simulink model "rigid_body_fdyn_rotmat_test_com"  (Simulink 8.5)
settings: Solver=ode4  StartTime=0.0  StopTime=0.01  FixedStep=1.000000e-04  RelTol=1e-3
undefined symbols (not defined in the file or in its folder): g_W, I_B_C, m, r_B_B_C
undefined symbols (not defined in the file): DynPar1, KinPar_mdh
libraries: lib_rigid_body_dynamics x3, lib_rigid_body_kinematics x3, lib_transformations x2, vrlib x1
settings Model: Creator=schappler  LastModifiedBy=schappler
settings DataIOCC: LimitDataPoints=off  SaveFormat=StructureWithTime  SignalLoggingSaveFormat=Dataset
settings OptimizationCC: ExpressionDepthLimit=128
settings DebuggingCC: UnderspecifiedInitializationDetection=Simplified  MergeDetectMultiDrivingBlocksExec=error  FcnCallInpInsideContextMsg=EnableAllAsError  StateNameClashWarn=none
settings GRTTargetCC: CombineOutputUpdateFcns=on  GRTInterface=off

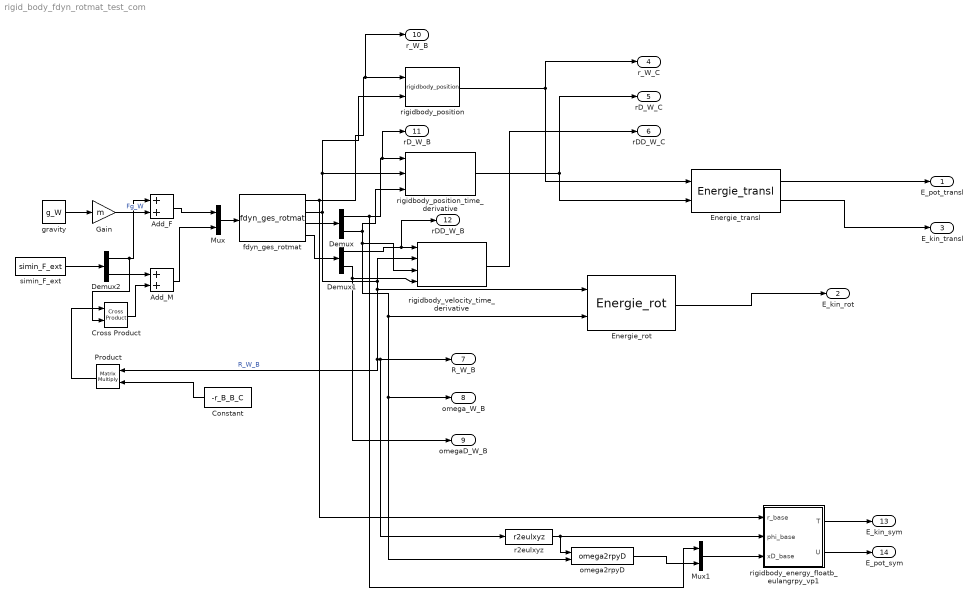
== system rigid_body_fdyn_rotmat_test_com ==
  Add_F : Sum
  Add_M : Sum
  Constant : Constant  Value=-r_B_B_C
  Cross Product : vrlib/Utilities/Cross Product
  Demux : Demux  Outputs=[3 3]
  Demux1 : Demux  Outputs=[3 3]
  Demux2 : Demux  Outputs=[3 3]
  Energie_rot : lib_rigid_body_dynamics/Energie_rot  I_B_C=I_B_C
  Energie_transl : lib_rigid_body_dynamics/Energie_transl  m=m  g_W=g_W
  Gain : Gain  Gain=m
  Mux : Mux  Inputs=2
  Mux1 : Mux  Inputs=2
  Product : Product  Multiplication=Matrix(*)
  r2eulxyz : lib_transformations/r2eulxyz
  fdyn_ges_rotmat : lib_rigid_body_dynamics/fdyn_ges_rotmat  I=I_B_C  m=m  r0=r0  rD0=rD0  R_t0=R_W_B_t0  omega0_t0=omega0_t0  r_B_B_C=r_B_B_C
  gravity : Constant  Value=g_W
  omega2rpyD : lib_transformations/omega2rpyD
  rigidbody_energy_floatb_eulangrpy_vp1 : Subsystem  mask{KinPar_mdh=KinPar_mdh, DynPar1=DynPar1, g_world=g_W}
      mask prompts: KinPar_mdh "Kinematik-Parameter"; DynPar1 "Dynamik-Parameter (Parametersatz 1)"; g_world "Gravitationsvektor im Welt-KS (g_world)"
  rigidbody_position : lib_rigid_body_kinematics/rigidbody_position  r_B_B_C=r_B_B_C  PktName_B='B'  PktName_C='C'
  rigidbody_position_time_derivative : lib_rigid_body_kinematics/rigidbody_position_time_derivative  r_B_B_C=r_B_B_C  PktName_B='B'  PktName_C='C'
  rigidbody_velocity_time_derivative : lib_rigid_body_kinematics/rigidbody_velocity_time_derivative  r_B_B_C=r_B_B_C  PktName_B='B'  PktName_C='C'
  simin_F_ext : FromWorkspace  VariableName=simin_F_ext  SampleTime=0  Interpolate=off  OutputAfterFinalValue=Holding final value
  E_pot_transl : Outport
  E_kin_rot : Outport  Port=2
  E_kin_transl : Outport  Port=3
  r_W_C : Outport  Port=4
  rD_W_C : Outport  Port=5
  rDD_W_C : Outport  Port=6
  R_W_B : Outport  Port=7
  omega_W_B : Outport  Port=8
  omegaD_W_B : Outport  Port=9
  r_W_B : Outport  Port=10
  rD_W_B : Outport  Port=11
  rDD_W_B : Outport  Port=12
  E_kin_sym : Outport  Port=13
  E_pot_sym : Outport  Port=14
  wires:
  gravity/1 -> Gain/1
  fdyn_ges_rotmat/2 -> rigidbody_position_time_derivative/2, rigidbody_position/2, rigidbody_velocity_time_derivative/2, Energie_rot/1, Product/1, r2eulxyz/1, R_W_B/1  "R_W_B"
  rigidbody_position/1 -> Energie_transl/1, r_W_C/1
  rigidbody_position_time_derivative/1 -> Energie_transl/2, rD_W_C/1
  Demux/2 -> rigidbody_position_time_derivative/3, rigidbody_velocity_time_derivative/3, Energie_rot/2, omega2rpyD/2, omega_W_B/1
  rigidbody_velocity_time_derivative/1 -> rDD_W_C/1
  Demux1/2 -> rigidbody_velocity_time_derivative/4, omegaD_W_B/1
  Energie_transl/1 -> E_pot_transl/1
  Energie_transl/2 -> E_kin_transl/1
  Energie_rot/1 -> E_kin_rot/1
  Gain/1 -> Add_F/2  "Fg_W"
  Mux/1 -> fdyn_ges_rotmat/1
  fdyn_ges_rotmat/3 -> Demux/1
  fdyn_ges_rotmat/1 -> rigidbody_energy_floatb_eulangrpy_vp1/1(r_base), rigidbody_position/1, r_W_B/1
  Demux/1 -> Mux1/1, rD_W_B/1, rigidbody_position_time_derivative/1
  fdyn_ges_rotmat/4 -> Demux1/1
  Demux1/1 -> rDD_W_B/1, rigidbody_velocity_time_derivative/1
  rigidbody_energy_floatb_eulangrpy_vp1/1(T) -> E_kin_sym/1
  rigidbody_energy_floatb_eulangrpy_vp1/2(U) -> E_pot_sym/1
  r2eulxyz/1 -> omega2rpyD/1, rigidbody_energy_floatb_eulangrpy_vp1/2(phi_base)
  omega2rpyD/1 -> Mux1/2
  Mux1/1 -> rigidbody_energy_floatb_eulangrpy_vp1/3(xD_base)
  simin_F_ext/1 -> Demux2/1
  Demux2/1 -> Cross Product/2, Add_F/1
  Demux2/2 -> Add_M/1
  Add_F/1 -> Mux/1
  Constant/1 -> Product/2
  Product/1 -> Cross Product/1
  Cross Product/1 -> Add_M/2
  Add_M/1 -> Mux/2

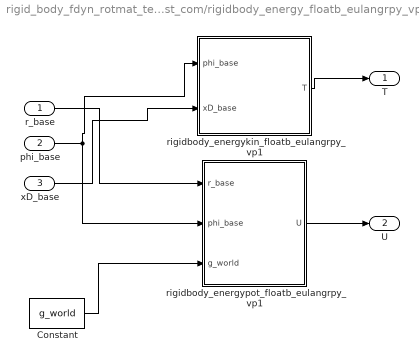
== system rigid_body_fdyn_rotmat_test_com/rigidbody_energy_floatb_eulangrpy_vp1 ==
  r_base : Inport
  phi_base : Inport  Port=2
  xD_base : Inport  Port=3
  Constant : Constant  Value=g_world
  rigidbody_energykin_floatb_eulangrpy_vp1 : Subsystem  mask{KinPar_mdh=KinPar_mdh, DynPar1=DynPar1}
      mask prompts: KinPar_mdh "Kinematik-Parameter"; DynPar1 "Dynamik-Parameter (Parametersatz 1)"
      mask init:
      | a_mdh = KinPar_mdh.a;
      | d_mdh = KinPar_mdh.d;
      | b_mdh = KinPar_mdh.b;
      | beta_mdh = KinPar_mdh.beta;
      | alpha_mdh = KinPar_mdh.alpha;
      | q_offset_mdh = KinPar_mdh.q_offset;
      | 
      | m = DynPar1.m;
      | r_S = DynPar1.r_S;
      | I_S = DynPar1.I_S;
  rigidbody_energypot_floatb_eulangrpy_vp1 : Subsystem  mask{KinPar_mdh=KinPar_mdh, DynPar1=DynPar1}
      mask prompts: KinPar_mdh "Kinematik-Parameter"; DynPar1 "Dynamik-Parameter (Parametersatz 1)"
      mask init: same as rigid_body_fdyn_rotmat_test_com/rigidbody_energy_floatb_eulangrpy_vp1/rigidbody_energykin_floatb_eulangrpy_vp1
  T : Outport
  U : Outport  Port=2
  wires:
  Constant/1 -> rigidbody_energypot_floatb_eulangrpy_vp1/3(g_world)
  rigidbody_energypot_floatb_eulangrpy_vp1/1(U) -> U/1
  rigidbody_energykin_floatb_eulangrpy_vp1/1(T) -> T/1
  phi_base/1 -> rigidbody_energykin_floatb_eulangrpy_vp1/1(phi_base), rigidbody_energypot_floatb_eulangrpy_vp1/2(phi_base)
  r_base/1 -> rigidbody_energypot_floatb_eulangrpy_vp1/1(r_base)
  xD_base/1 -> rigidbody_energykin_floatb_eulangrpy_vp1/2(xD_base)

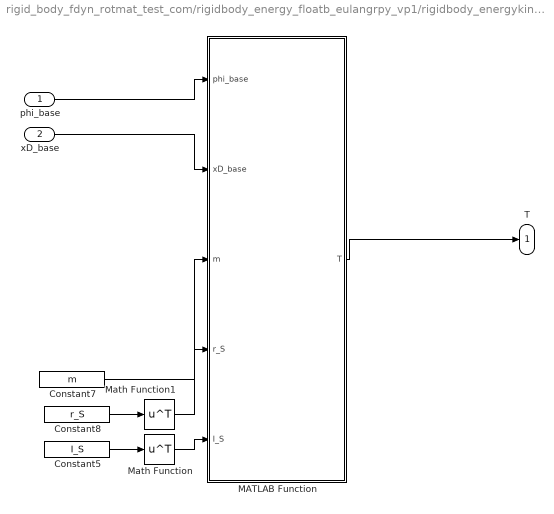
== system rigid_body_fdyn_rotmat_test_com/rigidbody_energy_floatb_eulangrpy_vp1/rigidbody_energykin_floatb_eulangrpy_vp1 ==
  phi_base : Inport
  xD_base : Inport  Port=2
  Constant5 : Constant  Value=I_S
  Constant7 : Constant  Value=m
  Constant8 : Constant  Value=r_S
  MATLAB Function : MATLAB Function  TreatAsAtomicUnit=on
  Math Function : Math  Operator=transpose  SaturateOnIntegerOverflow=on
  Math Function1 : Math  Operator=transpose  SaturateOnIntegerOverflow=on
  T : Outport
  wires:
  xD_base/1 -> MATLAB Function/2(xD_base)
  phi_base/1 -> MATLAB Function/1(phi_base)
  Constant5/1 -> Math Function/1
  Constant8/1 -> Math Function1/1
  Constant7/1 -> MATLAB Function/3(m)
  MATLAB Function/1(T) -> T/1
  Math Function/1 -> MATLAB Function/5(I_S)
  Math Function1/1 -> MATLAB Function/4(r_S)

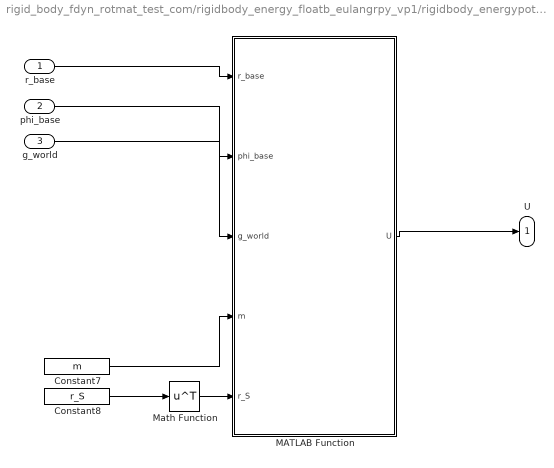
== system rigid_body_fdyn_rotmat_test_com/rigidbody_energy_floatb_eulangrpy_vp1/rigidbody_energypot_floatb_eulangrpy_vp1 ==
  r_base : Inport
  phi_base : Inport  Port=2
  g_world : Inport  Port=3
  Constant7 : Constant  Value=m
  Constant8 : Constant  Value=r_S
  MATLAB Function : MATLAB Function  TreatAsAtomicUnit=on
  Math Function : Math  Operator=transpose  SaturateOnIntegerOverflow=on
  U : Outport
  wires:
  phi_base/1 -> MATLAB Function/2(phi_base)
  r_base/1 -> MATLAB Function/1(r_base)
  Constant8/1 -> Math Function/1
  Constant7/1 -> MATLAB Function/4(m)
  g_world/1 -> MATLAB Function/3(g_world)
  MATLAB Function/1(U) -> U/1
  Math Function/1 -> MATLAB Function/5(r_S)

== matlab function rigidbody_energy_floatb_eulangrpy_vp1/rigidbody_energypot_floatb_eulangrpy_vp1/MATLAB Function ==
  data: U output double; r_base input double; phi_base input double; g_world input double; m input double; r_S input double
function U = energypot(r_base, phi_base, g_world, ...
  m, r_S)

q = zeros(0,1);
alpha_mdh = zeros(0,1);
a_mdh = zeros(0,1);
d_mdh = zeros(0,1);
q_offset_mdh = zeros(0,1);
b_mdh = zeros(0,1);
beta_mdh = zeros(0,1);

%#codegen
U = rigidbody_energypot_floatb_eulangrpy_slag_vp1(q, r_base, phi_base, g_world, ...
  alpha_mdh, a_mdh, d_mdh, q_offset_mdh, b_mdh, beta_mdh, m, r_S);

== matlab function rigidbody_energy_floatb_eulangrpy_vp1/rigidbody_energykin_floatb_eulangrpy_vp1/MATLAB Function ==
  data: T output double; phi_base input double; xD_base input double; m input double; r_S input double; I_S input double
function T = energykin(phi_base, xD_base,  ...
  m, r_S, I_S)

q = zeros(0,1);
qD = zeros(0,1);
alpha_mdh = zeros(0,1);
a_mdh = zeros(0,1);
d_mdh = zeros(0,1);
q_offset_mdh = zeros(0,1);
b_mdh = zeros(0,1);
beta_mdh = zeros(0,1);

%#codegen
T = rigidbody_energykin_floatb_eulangrpy_slag_vp1(q, qD, phi_base, xD_base, ...
  alpha_mdh, a_mdh, d_mdh, q_offset_mdh, b_mdh, beta_mdh, m, r_S, I_S);
